simulink model "DeliveryDroneArchitecture"  (R2024a)
settings: Solver=VariableStepAuto  StartTime=0.0  StopTime=10.0  RelTol=1e-3
settings Model: Creator=callie  LastModifiedBy=callie

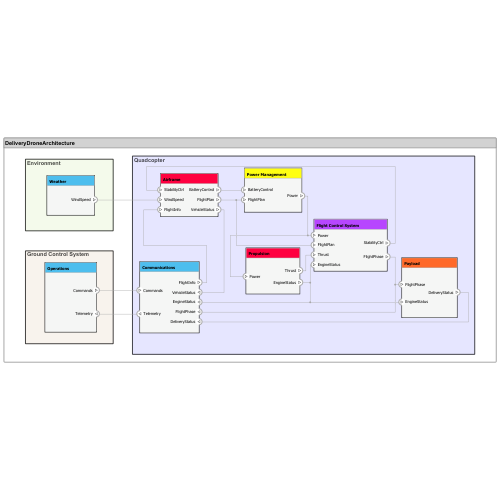
[thumbnail: Simulink's stored preview of the top-level diagram]
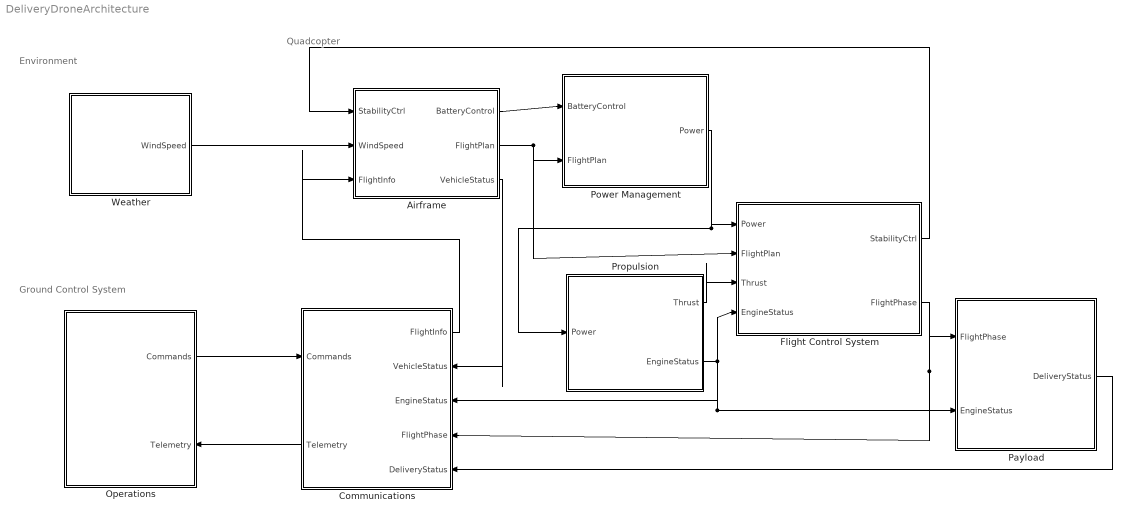
== system DeliveryDroneArchitecture ==
  note: Quadcopter
  note: Ground Control System
  note: Environment
  Airframe : Subsystem
      settings: PortSchema="{\"entries\":[{\"content\":{\"headerSize\":26,\"margin\":15,\"minimumSpacing\":25,\"sides\":[{\"content\":{\"connectorIds\":[\"In1\",\"In2\",\"In3\"]},\"type\":\"ConnectorPlacement.EquallySpacedRectSide\",\"uuid\":\"6da6e52a-0990-40db-aa67-08a7a38817fa\"},{\"content\":{\"connectorIds\":[\"Out1\",\"Out2\",\"Out3\"],\"side\":\"RIGHT\"},\"type\":\"ConnectorPlacement.EquallySpacedRectSide\",\"uuid\":\"269c5b85-9bbc-44b1-804d-a8d590ef4faf\"},{\"content\":{\"side\":\"TOP\"},\"type\":\"ConnectorPlacement.EquallySpacedRectSide\",\"uuid\":\"fc7a0441-689a-498e-9011-17f79e270a3a\"}]},\"type\":\"ConnectorPlacement.EquallySpacedConnector\",\"uuid\":\"cc86e059-7bec-45b6-8e55-861330b424d3\"}],\"packageUris\":[\"http://schema.mathworks.com/mf0/Connector/R2020b\"],\"version\":\"1.0\"}"
  Communications : Subsystem
      settings: PortSchema="{\"entries\":[{\"content\":{\"headerSize\":26,\"margin\":15,\"minimumSpacing\":25,\"sides\":[{\"content\":{\"connectorIds\":[\"In3\",\"Out2\"]},\"type\":\"ConnectorPlacement.EquallySpacedRectSide\",\"uuid\":\"6da6e52a-0990-40db-aa67-08a7a38817fa\"},{\"content\":{\"connectorIds\":[\"Out1\",\"In5\",\"In1\",\"In2\",\"In4\"],\"side\":\"RIGHT\"},\"type\":\"ConnectorPlacement.EquallySpacedRectSide\",\"uuid\":\"269c5b85-9bbc-44b1-804d-a8d590ef4faf\"},{\"content\":{\"side\":\"TOP\"},\"type\":\"ConnectorPlacement.EquallySpacedRectSide\",\"uuid\":\"fc7a0441-689a-498e-9011-17f79e270a3a\"}]},\"type\":\"ConnectorPlacement.EquallySpacedConnector\",\"uuid\":\"cc86e059-7bec-45b6-8e55-861330b424d3\"}],\"packageUris\":[\"http://schema.mathworks.com/mf0/Connector/R2020b\"],\"version\":\"1.0\"}"
  Flight Control System : Subsystem
      settings: PortSchema="{\"entries\":[{\"content\":{\"headerSize\":26,\"margin\":15,\"minimumSpacing\":25,\"sides\":[{\"content\":{\"connectorIds\":[\"In2\",\"In1\",\"In3\",\"In4\"]},\"type\":\"ConnectorPlacement.EquallySpacedRectSide\",\"uuid\":\"6da6e52a-0990-40db-aa67-08a7a38817fa\"},{\"content\":{\"connectorIds\":[\"Out1\",\"Out2\"],\"side\":\"RIGHT\"},\"type\":\"ConnectorPlacement.EquallySpacedRectSide\",\"uuid\":\"269c5b85-9bbc-44b1-804d-a8d590ef4faf\"},{\"content\":{\"side\":\"TOP\"},\"type\":\"ConnectorPlacement.EquallySpacedRectSide\",\"uuid\":\"fc7a0441-689a-498e-9011-17f79e270a3a\"}]},\"type\":\"ConnectorPlacement.EquallySpacedConnector\",\"uuid\":\"cc86e059-7bec-45b6-8e55-861330b424d3\"}],\"packageUris\":[\"http://schema.mathworks.com/mf0/Connector/R2020b\"],\"version\":\"1.0\"}"
  Operations : Subsystem
      settings: PortSchema="{\"entries\":[{\"content\":{\"headerSize\":26,\"margin\":15,\"minimumSpacing\":25,\"sides\":[{\"content\":{},\"type\":\"ConnectorPlacement.EquallySpacedRectSide\",\"uuid\":\"6da6e52a-0990-40db-aa67-08a7a38817fa\"},{\"content\":{\"connectorIds\":[\"Out1\",\"In1\"],\"side\":\"RIGHT\"},\"type\":\"ConnectorPlacement.EquallySpacedRectSide\",\"uuid\":\"269c5b85-9bbc-44b1-804d-a8d590ef4faf\"},{\"content\":{\"side\":\"TOP\"},\"type\":\"ConnectorPlacement.EquallySpacedRectSide\",\"uuid\":\"fc7a0441-689a-498e-9011-17f79e270a3a\"}]},\"type\":\"ConnectorPlacement.EquallySpacedConnector\",\"uuid\":\"cc86e059-7bec-45b6-8e55-861330b424d3\"}],\"packageUris\":[\"http://schema.mathworks.com/mf0/Connector/R2020b\"],\"version\":\"1.0\"}"
  "Payload " : Subsystem
      settings: PortSchema="{\"entries\":[{\"content\":{\"headerSize\":26,\"margin\":15,\"minimumSpacing\":25,\"sides\":[{\"content\":{\"connectorIds\":[\"In1\",\"In2\"]},\"type\":\"ConnectorPlacement.EquallySpacedRectSide\",\"uuid\":\"6da6e52a-0990-40db-aa67-08a7a38817fa\"},{\"content\":{\"connectorIds\":[\"Out1\"],\"side\":\"RIGHT\"},\"type\":\"ConnectorPlacement.EquallySpacedRectSide\",\"uuid\":\"269c5b85-9bbc-44b1-804d-a8d590ef4faf\"},{\"content\":{\"side\":\"TOP\"},\"type\":\"ConnectorPlacement.EquallySpacedRectSide\",\"uuid\":\"fc7a0441-689a-498e-9011-17f79e270a3a\"}]},\"type\":\"ConnectorPlacement.EquallySpacedConnector\",\"uuid\":\"cc86e059-7bec-45b6-8e55-861330b424d3\"}],\"packageUris\":[\"http://schema.mathworks.com/mf0/Connector/R2020b\"],\"version\":\"1.0\"}"
  Power Management : Subsystem
      settings: PortSchema="{\"entries\":[{\"content\":{\"headerSize\":26,\"margin\":15,\"minimumSpacing\":25,\"sides\":[{\"content\":{\"connectorIds\":[\"In1\",\"In2\"]},\"type\":\"ConnectorPlacement.EquallySpacedRectSide\",\"uuid\":\"6da6e52a-0990-40db-aa67-08a7a38817fa\"},{\"content\":{\"connectorIds\":[\"Out1\"],\"side\":\"RIGHT\"},\"type\":\"ConnectorPlacement.EquallySpacedRectSide\",\"uuid\":\"269c5b85-9bbc-44b1-804d-a8d590ef4faf\"},{\"content\":{\"side\":\"TOP\"},\"type\":\"ConnectorPlacement.EquallySpacedRectSide\",\"uuid\":\"fc7a0441-689a-498e-9011-17f79e270a3a\"}]},\"type\":\"ConnectorPlacement.EquallySpacedConnector\",\"uuid\":\"cc86e059-7bec-45b6-8e55-861330b424d3\"}],\"packageUris\":[\"http://schema.mathworks.com/mf0/Connector/R2020b\"],\"version\":\"1.0\"}"
  Propulsion : Subsystem
      settings: PortSchema="{\"entries\":[{\"content\":{\"headerSize\":26,\"margin\":15,\"minimumSpacing\":25,\"sides\":[{\"content\":{\"connectorIds\":[\"In1\"]},\"type\":\"ConnectorPlacement.EquallySpacedRectSide\",\"uuid\":\"6da6e52a-0990-40db-aa67-08a7a38817fa\"},{\"content\":{\"connectorIds\":[\"Out2\",\"Out1\"],\"side\":\"RIGHT\"},\"type\":\"ConnectorPlacement.EquallySpacedRectSide\",\"uuid\":\"269c5b85-9bbc-44b1-804d-a8d590ef4faf\"},{\"content\":{\"side\":\"TOP\"},\"type\":\"ConnectorPlacement.EquallySpacedRectSide\",\"uuid\":\"fc7a0441-689a-498e-9011-17f79e270a3a\"}]},\"type\":\"ConnectorPlacement.EquallySpacedConnector\",\"uuid\":\"cc86e059-7bec-45b6-8e55-861330b424d3\"}],\"packageUris\":[\"http://schema.mathworks.com/mf0/Connector/R2020b\"],\"version\":\"1.0\"}"
  Weather : Subsystem
      settings: PortSchema="{\"entries\":[{\"content\":{\"headerSize\":26,\"margin\":15,\"minimumSpacing\":25,\"sides\":[{\"content\":{},\"type\":\"ConnectorPlacement.EquallySpacedRectSide\",\"uuid\":\"6da6e52a-0990-40db-aa67-08a7a38817fa\"},{\"content\":{\"connectorIds\":[\"Out1\"],\"side\":\"RIGHT\"},\"type\":\"ConnectorPlacement.EquallySpacedRectSide\",\"uuid\":\"269c5b85-9bbc-44b1-804d-a8d590ef4faf\"},{\"content\":{\"side\":\"TOP\"},\"type\":\"ConnectorPlacement.EquallySpacedRectSide\",\"uuid\":\"fc7a0441-689a-498e-9011-17f79e270a3a\"}]},\"type\":\"ConnectorPlacement.EquallySpacedConnector\",\"uuid\":\"cc86e059-7bec-45b6-8e55-861330b424d3\"}],\"packageUris\":[\"http://schema.mathworks.com/mf0/Connector/R2020b\"],\"version\":\"1.0\"}"
  wires:
  Communications/2(Telemetry) -> Operations/1(Telemetry)
  Operations/1(Commands) -> Communications/3(Commands)
  Weather/1(WindSpeed) -> Airframe/2(WindSpeed)
  Airframe/1(BatteryControl) -> Power Management/1(BatteryControl)
  Communications/1(FlightInfo) -> Airframe/3(FlightInfo)
  Airframe/3(VehicleStatus) -> Communications/5(VehicleStatus)
  Power Management/1(Power) -> Flight Control System/2(Power), Propulsion/1(Power)
  Propulsion/2(Thrust) -> Flight Control System/3(Thrust)
  Propulsion/1(EngineStatus) -> Communications/1(EngineStatus), "Payload "/2(EngineStatus), Flight Control System/4(EngineStatus)
  Flight Control System/2(FlightPhase) -> Communications/2(FlightPhase), "Payload "/1(FlightPhase)
  "Payload "/1(DeliveryStatus) -> Communications/4(DeliveryStatus)
  Airframe/2(FlightPlan) -> Flight Control System/1(FlightPlan), Power Management/2(FlightPlan)
  Flight Control System/1(StabilityCtrl) -> Airframe/1(StabilityCtrl)

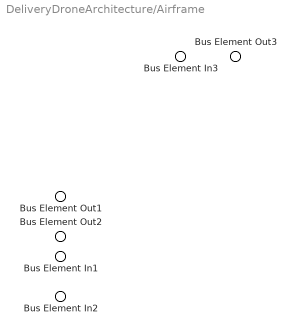
== system DeliveryDroneArchitecture/Airframe ==
  Bus Element In3 : Inport  PortName=StabilityCtrl
  Bus Element In1 : Inport  Port=2  PortName=WindSpeed
  Bus Element In2 : Inport  Port=3  PortName=FlightInfo
  Bus Element Out1 : Outport  PortName=BatteryControl
  Bus Element Out3 : Outport  Port=2  PortName=FlightPlan
  Bus Element Out2 : Outport  Port=3  PortName=VehicleStatus

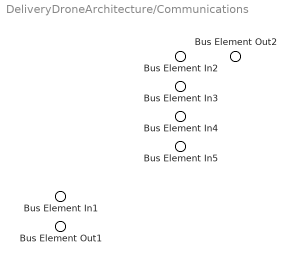
== system DeliveryDroneArchitecture/Communications ==
  Bus Element In5 : Inport  PortName=EngineStatus
  Bus Element In4 : Inport  Port=2  PortName=FlightPhase
  Bus Element In2 : Inport  Port=3  PortName=Commands
  Bus Element In3 : Inport  Port=4  PortName=DeliveryStatus
  Bus Element In1 : Inport  Port=5  PortName=VehicleStatus
  Bus Element Out2 : Outport  PortName=FlightInfo
  Bus Element Out1 : Outport  Port=2  PortName=Telemetry

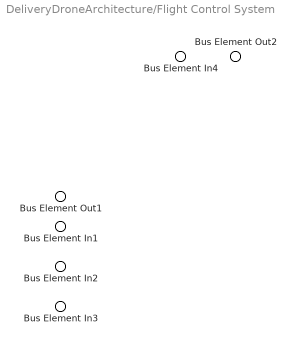
== system DeliveryDroneArchitecture/Flight Control System ==
  Bus Element In4 : Inport  PortName=FlightPlan
  Bus Element In1 : Inport  Port=2  PortName=Power
  Bus Element In2 : Inport  Port=3  PortName=Thrust
  Bus Element In3 : Inport  Port=4  PortName=EngineStatus
  Bus Element Out2 : Outport  PortName=StabilityCtrl
  Bus Element Out1 : Outport  Port=2  PortName=FlightPhase

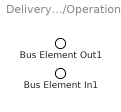
== system DeliveryDroneArchitecture/Operations ==
  Bus Element In1 : Inport  PortName=Telemetry
  Bus Element Out1 : Outport  PortName=Commands

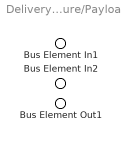
== system DeliveryDroneArchitecture/Payload  ==
  Bus Element In1 : Inport  PortName=FlightPhase
  Bus Element In2 : Inport  Port=2  PortName=EngineStatus
  Bus Element Out1 : Outport  PortName=DeliveryStatus

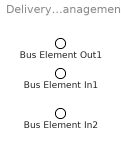
== system DeliveryDroneArchitecture/Power Management ==
  Bus Element In1 : Inport  PortName=BatteryControl
  Bus Element In2 : Inport  Port=2  PortName=FlightPlan
  Bus Element Out1 : Outport  PortName=Power

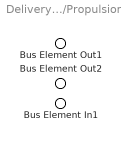
== system DeliveryDroneArchitecture/Propulsion ==
  Bus Element In1 : Inport  PortName=Power
  Bus Element Out1 : Outport  PortName=EngineStatus
  Bus Element Out2 : Outport  Port=2  PortName=Thrust

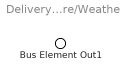
== system DeliveryDroneArchitecture/Weather ==
  Bus Element Out1 : Outport  PortName=WindSpeed
